simulink model "NNController_SCARA"  (R2023b)
settings: Solver=VariableStepAuto  StartTime=0.0  StopTime=30  RelTol=1e-3
settings Model: Creator=Hamid Reza  LastModifiedBy=Hamid Reza

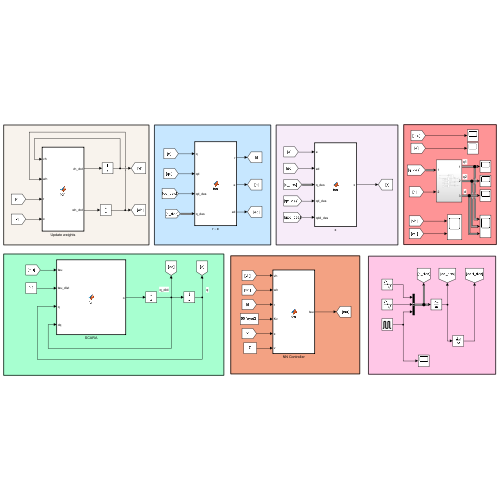
[thumbnail: Simulink's stored preview of the top-level diagram]
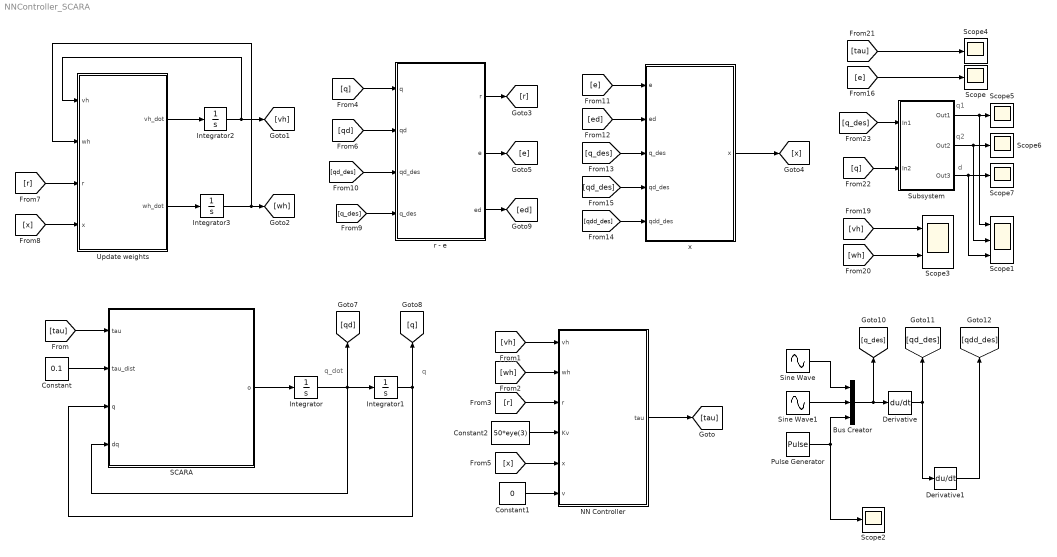
== system NNController_SCARA ==
  note: q_dot
  note: q
  note: q2
  note: d
  note: q1
  Bus Creator : BusCreator  Inputs=3
  Constant : Constant  Value=0.1
  Constant1 : Constant  Value=0
  Constant2 : Constant  Value=50*eye(3)
  Derivative : Derivative
  Derivative1 : Derivative
  Integrator : Integrator  InitialCondition=zeros(3,1)
  Integrator1 : Integrator  InitialCondition=zeros(3,1)
  Integrator2 : Integrator  InitialCondition=zeros(15,5)
  Integrator3 : Integrator  InitialCondition=zeros(5,3)
  NN Controller : MATLAB Function  TreatAsAtomicUnit=on
  Pulse Generator : DiscretePulseGenerator  PulseType=Time based  Period=5  PulseWidth=50
  SCARA : MATLAB Function  TreatAsAtomicUnit=on
  Scope{,2,4..7} (6 alike) : Scope
  Scope1 : Scope  NumInputPorts=3
  Scope3 : Scope  NumInputPorts=2
  Sine Wave : Sin  Frequency=2  SampleTime=0
  Sine Wave1 : Sin  Frequency=2  Phase=pi/2  SampleTime=0
  Subsystem : Subsystem
  Update weights : MATLAB Function  TreatAsAtomicUnit=on
  r - e : MATLAB Function  TreatAsAtomicUnit=on
  x : MATLAB Function  TreatAsAtomicUnit=on
  wires:
  Integrator1/1 -> SCARA/3(q), [q]
  SCARA/1(o) -> Integrator/1
  Integrator/1 -> SCARA/4(dq), Integrator1/1, [qd]
  Constant/1 -> SCARA/2(tau_dist)
  [tau] -> SCARA/1(tau)
  NN Controller/1(tau) -> [tau]
  [vh] -> NN Controller/1(vh)
  [wh] -> NN Controller/2(wh)
  [r] -> NN Controller/3(r)
  Constant2/1 -> NN Controller/4(Kv)
  [x] -> NN Controller/5(x)
  Constant1/1 -> NN Controller/6(v)
  Integrator2/1 -> [vh], Update weights/1(vh)
  [x] -> Update weights/4(x)
  [r] -> Update weights/3(r)
  Update weights/1(vh_dot) -> Integrator2/1
  Update weights/2(wh_dot) -> Integrator3/1
  Integrator3/1 -> Update weights/2(wh), [wh]
  [q] -> r - e/1(q)
  [qd] -> r - e/2(qd)
  [q_des] -> r - e/4(q_des)
  [qd_des] -> x/4(qd_des)
  [e] -> x/1(e)
  [qdd_des] -> x/5(qdd_des)
  x/1(x) -> [x]
  [ed] -> x/2(ed)
  [q_des] -> x/3(q_des)
  r - e/1(r) -> [r]
  r - e/2(e) -> [e]
  [qd_des] -> r - e/3(qd_des)
  r - e/3(ed) -> [ed]
  Sine Wave/1 -> Bus Creator/1
  Sine Wave1/1 -> Bus Creator/2
  Bus Creator/1 -> [q_des], Derivative/1
  Derivative/1 -> Derivative1/1, [qd_des]
  Derivative1/1 -> [qdd_des]
  Pulse Generator/1 -> Bus Creator/3, Scope2/1
  [e] -> Scope/1
  [wh] -> Scope3/2
  [vh] -> Scope3/1
  [tau] -> Scope4/1
  [q_des] -> Subsystem/1(In1)
  [q] -> Subsystem/2(In2)
  Subsystem/1(Out1) -> Scope1/1, Scope5/1
  Subsystem/2(Out2) -> Scope1/2, Scope6/1
  Subsystem/3(Out3) -> Scope1/3, Scope7/1

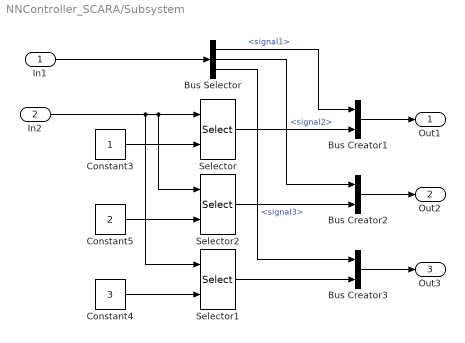
== system NNController_SCARA/Subsystem ==
  In1 : Inport
  In2 : Inport  Port=2
  Bus Creator1 : BusCreator  Inputs=2
  Bus Creator2 : BusCreator  Inputs=2
  Bus Creator3 : BusCreator  Inputs=2
  Bus Selector : BusSelector  OutputSignals=signal1,signal2,signal3
  Constant3 : Constant
  Constant4 : Constant  Value=3
  Constant5 : Constant  Value=2
  Selector : Selector  InputPortWidth=3  IndexOptions=Index vector (port)  Indices=1  OutputSizes=1
  Selector1 : Selector  InputPortWidth=3  IndexOptions=Index vector (port)  Indices=1  OutputSizes=1
  Selector2 : Selector  InputPortWidth=3  IndexOptions=Index vector (port)  Indices=1  OutputSizes=1
  Out1 : Outport
  Out2 : Outport  Port=2
  Out3 : Outport  Port=3
  wires:
  Bus Selector/3 -> Bus Creator3/1  "<signal3>"
  Bus Selector/2 -> Bus Creator2/1  "<signal2>"
  Selector2/1 -> Bus Creator2/2
  Constant3/1 -> Selector/2
  Selector/1 -> Bus Creator1/2
  Bus Selector/1 -> Bus Creator1/1  "<signal1>"
  Bus Creator3/1 -> Out3/1
  Selector1/1 -> Bus Creator3/2
  Constant5/1 -> Selector2/2
  Constant4/1 -> Selector1/2
  In2/1 -> Selector1/1, Selector2/1, Selector/1
  Bus Creator2/1 -> Out2/1
  Bus Creator1/1 -> Out1/1
  In1/1 -> Bus Selector/1

== matlab function NNController_SCARA/NN Controller ==
  data: vh input; tau output; wh input; r input; Kv input; x input; v input
function tau = fcn(vh,wh,r,Kv,x,v)
sigma = 1./(1.+exp(-vh'*x));
tau = wh'*sigma + Kv*r - v;

== matlab function NNController_SCARA/SCARA ==
  data: tau input; tau_dist input; q input; dq input; o output
function o  = fcn(tau,tau_dist,q,dq)



theta1=q(1);
theta2=q(2);
d=q(3);

dtheta1=dq(1);
dtheta2=dq(2);
dd=dq(3);


a1=0.6;
a2=0.4;
m1=12;
m2=6;
m3=6;
g = 9.81;


% define mass matrix

m11 = (1/3)*m1*a1^2+m2*(a1^2+(1/3)*a2^2+a1*a2*cos(theta2))+m3*(a1^2+a2^2+2*a1*a2*cos(theta2));
m12 = -m2*a2*((1/3)*a2+(1/2)*a1*cos(theta2))-m3*(a2^2+a1*a2*cos(theta2));
m13 = 0;
m21 = m12;
m22 = (1/3)*m2*a2^2+m3*(a2^2);
m23 = 0;
m31 = m13;
m32 = m23;
m33 = m3;

M = [m11,m12,m13;m21,m22,m23;m31,m32,m33];


% define gravity matrix

g = [0; 0; -m3*g];

% define coriolis and centrifugal matrix

c1 = -(m2+2*m3)*a1*a2*sin(theta2)*(dtheta1*dtheta2+((1/2)*dtheta2^2));
c2 = ((1/2)*m2+m3)*a1*a2*sin(theta2)*(dtheta1^2);
c3 = 0;

C = [c1 ; c2 ; c3];


o=pinv(M)*(tau+tau_dist-(C+g));

== matlab function NNController_SCARA/Update weights ==
  data: vh input; vh_dot output; wh input; r input; x input; wh_dot output
function [vh_dot, wh_dot] = fcn(vh,wh,r,x)


G = 20;
F = 30;

wh_dot = F*(1./(1.+exp(vh'*x))*r');
vh_dot = G*(x*(sigma_p(vh'*x)'*wh*r)');
end

function o = sigma_p(z)
sig = 1./(1.+exp(-z));
o = diag(sig.*(1.-sig));
end

== matlab function NNController_SCARA/r - e ==
  data: q input; r output; qd input; qd_des input; q_des input; e output; ed output
function [r,e,ed] = fcn(q,qd,qd_des,q_des)
e = q_des - q;
ed = qd_des - qd;

r = ed + 90*e;

== matlab function NNController_SCARA/x ==
  data: e input; x output; ed input; q_des input; qd_des input; qdd_des input
function x = fcn(e,ed,q_des,qd_des,qdd_des)
x = [e',ed',q_des',qd_des',qdd_des']';
